simulink model "constant_rv_envTest"  (R2018b)
settings: Solver=FixedStepAuto  StartTime=0.0  StopTime=120  RelTol=1e-3  EnableMultiTasking=on
undefined symbols (not defined in the file or in its folder): attitude_estimation_lib, fswParams, simParams, t0, triad_coarse_estimator, TRIAD_coarse_estimator
libraries: vrlib x8, dspmathops x6, aerolibutil x5, magField_lib x2, time_Lib x2, solarPressure_lib x1, clock_lib x1, eclipseCheck x1, sunVector_lib x1, extended_kalman_filter_lib x1
settings Model: Creator=devantormey  LastModifiedBy=devantormey
settings OptimizationCC: LifeSpan=inf
settings DebuggingCC: SFUnexpectedBacktrackingDiag=warning  SFNoUnconditionalDefaultTransitionDiag=warning
settings SFSimCC: SimUseLocalCustomCode=off
settings RTWCC: RTWUseLocalCustomCode=off
settings CodeAppCC: StateflowObjectComments=on
settings GRTTargetCC: TargetLangStandard=C89/C90 (ANSI)  GeneratePreprocessorConditionals=Disable all
settings ConfigComp: CovMetricSettings=dw  CovHtmlReporting=on  CovSaveCumulativeToWorkspaceVar=on  CovSaveSingleToWorkspaceVar=on  CovExternalEMLEnable=off

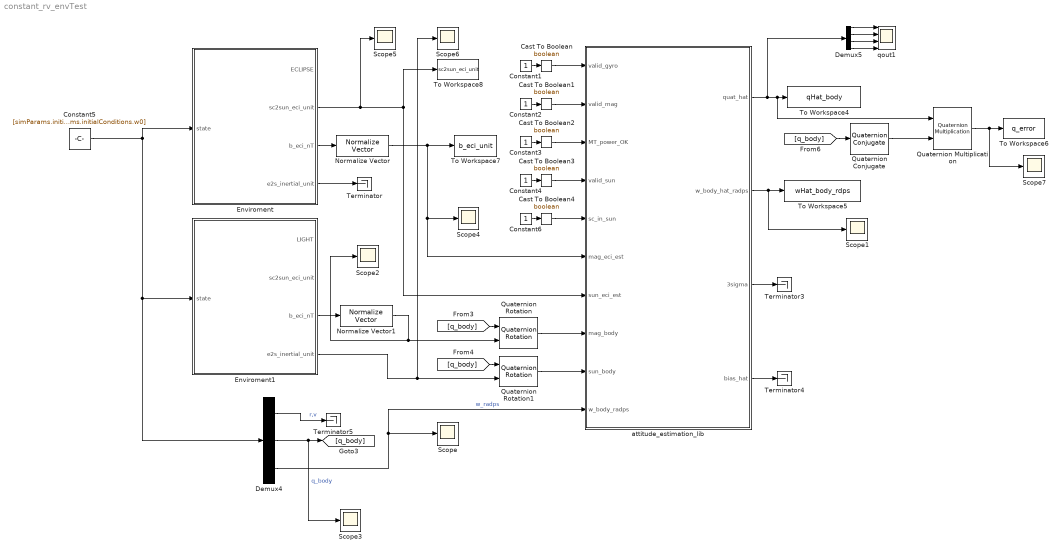
== system constant_rv_envTest ==
  Cast To Boolean{,1..4} (5 alike) : DataTypeConversion  OutDataTypeStr=boolean
  Constant{1..4,6} (5 alike) : Constant
  Constant5 : Constant  Value=[simParams.initialConditions.r0;simParams.initialConditions.v0;simParams.initialConditions.q0;simParams.initialConditions.w0]
  Demux4 : Demux  Outputs=[6 4 3]
  Demux5 : Demux
  Enviroment : Subsystem
  Enviroment1 : Subsystem
  Normalize Vector : vrlib/Utilities/Normalize Vector  maxzero=0
      settings: SourceProductName=Simulink 3D Animation  SourceProductBaseCode=VR
  Normalize Vector1 : vrlib/Utilities/Normalize Vector  maxzero=0
      settings: SourceProductName=Simulink 3D Animation  SourceProductBaseCode=VR
  Quaternion Conjugate : aerolibutil/Quaternion Conjugate
      settings: SourceProductName=Aerospace Blockset  SourceProductBaseCode=AE
  Quaternion Multiplication : aerolibutil/Quaternion Multiplication
  Quaternion Rotation : aerolibutil/Quaternion Rotation
  Quaternion Rotation1 : aerolibutil/Quaternion Rotation
  Scope{,1..7} (8 alike) : Scope
  Terminator{,3..5} (4 alike) : Terminator
  To Workspace4 : ToWorkspace  VariableName=qHat_body  SaveFormat=Timeseries  SampleTime=-1
  To Workspace5 : ToWorkspace  VariableName=wHat_body_rdps  SaveFormat=Timeseries  SampleTime=-1
  To Workspace6 : ToWorkspace  VariableName=q_error  SaveFormat=Timeseries  SampleTime=-1
  To Workspace7 : ToWorkspace  VariableName=b_eci_unit  SaveFormat=Timeseries  SampleTime=-1
  To Workspace8 : ToWorkspace  VariableName=sc2sun_eci_unit  SaveFormat=Timeseries  SampleTime=-1
  attitude_estimation_lib : Subsystem  AncestorBlock=attitude_estimation_lib/attitude_estimation_lib
  qout1 : Scope  NumInputPorts=4
  wires:
  attitude_estimation_lib/2(w_body_hat_radps) -> Scope1/1, To Workspace5/1
  attitude_estimation_lib/3(3sigma) -> Terminator3/1
  Constant1/1 -> Cast To Boolean/1
  Constant2/1 -> Cast To Boolean1/1
  Constant3/1 -> Cast To Boolean2/1
  Constant4/1 -> Cast To Boolean3/1
  Demux4/1 -> Terminator5/1  "r,v"
  Demux4/2 -> Scope3/1, [q_body]  "q_body"
  Normalize Vector1/1 -> Quaternion Rotation/2, Scope2/1
  [q_body] -> Quaternion Rotation/1
  [q_body] -> Quaternion Rotation1/1
  Enviroment1/4(e2s_inertial_unit) -> Quaternion Rotation1/2, Scope6/1
  Demux5/1 -> qout1/1
  Demux5/3 -> qout1/3
  Demux5/2 -> qout1/2
  Demux5/4 -> qout1/4
  Cast To Boolean/1 -> attitude_estimation_lib/1(valid_gyro)
  Cast To Boolean1/1 -> attitude_estimation_lib/2(valid_mag)
  Cast To Boolean2/1 -> attitude_estimation_lib/3(MT_power_OK)
  Cast To Boolean3/1 -> attitude_estimation_lib/4("valid_sun ")
  Cast To Boolean4/1 -> attitude_estimation_lib/5(sc_in_sun)
  Normalize Vector/1 -> Scope4/1, attitude_estimation_lib/6(mag_eci_est), To Workspace7/1
  Enviroment/2(sc2sun_eci_unit) -> Scope5/1, attitude_estimation_lib/7(sun_eci_est), To Workspace8/1
  Quaternion Rotation/1 -> attitude_estimation_lib/8(mag_body)
  Quaternion Rotation1/1 -> attitude_estimation_lib/9(sun_body)
  Demux4/3 -> attitude_estimation_lib/10(w_body_radps), Scope/1  "w_radps"
  attitude_estimation_lib/4(bias_hat) -> Terminator4/1
  attitude_estimation_lib/1(quat_hat) -> Demux5/1, Quaternion Multiplication/1, To Workspace4/1
  Enviroment/3(b_eci_nT) -> Normalize Vector/1
  Enviroment/4(e2s_inertial_unit) -> Terminator/1
  Quaternion Conjugate/1 -> Quaternion Multiplication/2
  [q_body] -> Quaternion Conjugate/1
  Quaternion Multiplication/1 -> Scope7/1, To Workspace6/1
  Enviroment1/3(b_eci_nT) -> Normalize Vector1/1
  Constant6/1 -> Cast To Boolean4/1
  Constant5/1 -> Demux4/1, Enviroment1/1(state), Enviroment/1(state)

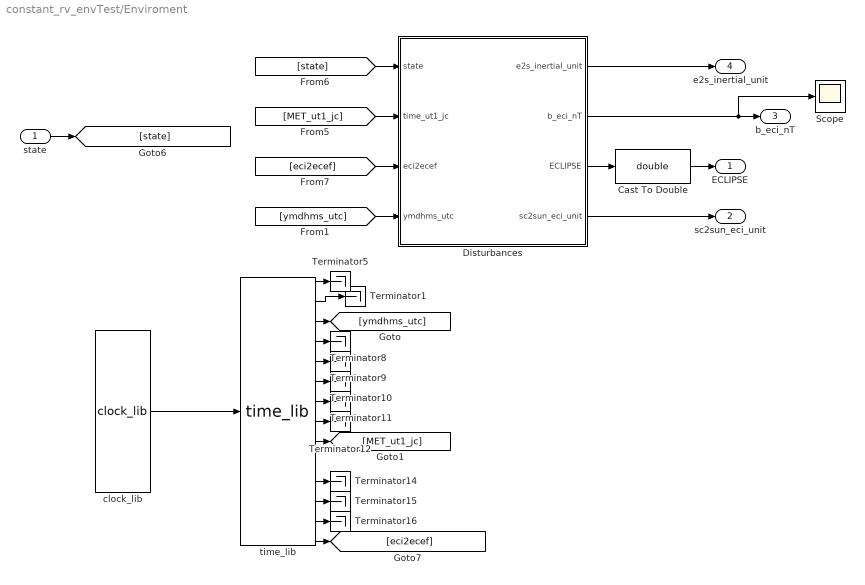
== system constant_rv_envTest/Enviroment ==
  state : Inport
  Cast To Double : DataTypeConversion  OutDataTypeStr=double
  Disturbances : Subsystem
  Scope : Scope
  Terminator{1,5,8..12,14..16} (10 alike) : Terminator
  clock_lib : clock_lib/clock_lib  SystemSampleTime=-1
  "time_lib " : time_Lib/time_lib    SystemSampleTime=-1
  ECLIPSE : Outport
  sc2sun_eci_unit : Outport  Port=2
  b_eci_nT : Outport  Port=3
  e2s_inertial_unit : Outport  Port=4
  wires:
  state/1 -> [state]
  clock_lib/1 -> "time_lib "/1
  "time_lib "/14 -> [eci2ecef]
  [eci2ecef] -> Disturbances/3(eci2ecef)
  [MET_ut1_jc] -> Disturbances/2(time_ut1_jc)
  [state] -> Disturbances/1(state)
  Cast To Double/1 -> ECLIPSE/1
  Disturbances/3(ECLIPSE) -> Cast To Double/1
  "time_lib "/1 -> Terminator5/1
  "time_lib "/2 -> Terminator1/1
  "time_lib "/3 -> [ymdhms_utc]
  "time_lib "/4 -> Terminator8/1
  "time_lib "/5 -> Terminator9/1
  "time_lib "/6 -> Terminator10/1
  "time_lib "/7 -> Terminator11/1
  "time_lib "/8 -> Terminator12/1
  "time_lib "/9 -> [MET_ut1_jc]
  "time_lib "/11 -> Terminator14/1
  "time_lib "/12 -> Terminator15/1
  "time_lib "/13 -> Terminator16/1
  [ymdhms_utc] -> Disturbances/4(ymdhms_utc)
  Disturbances/4(sc2sun_eci_unit) -> sc2sun_eci_unit/1
  Disturbances/2(b_eci_nT) -> Scope/1, b_eci_nT/1
  Disturbances/1(e2s_inertial_unit) -> e2s_inertial_unit/1

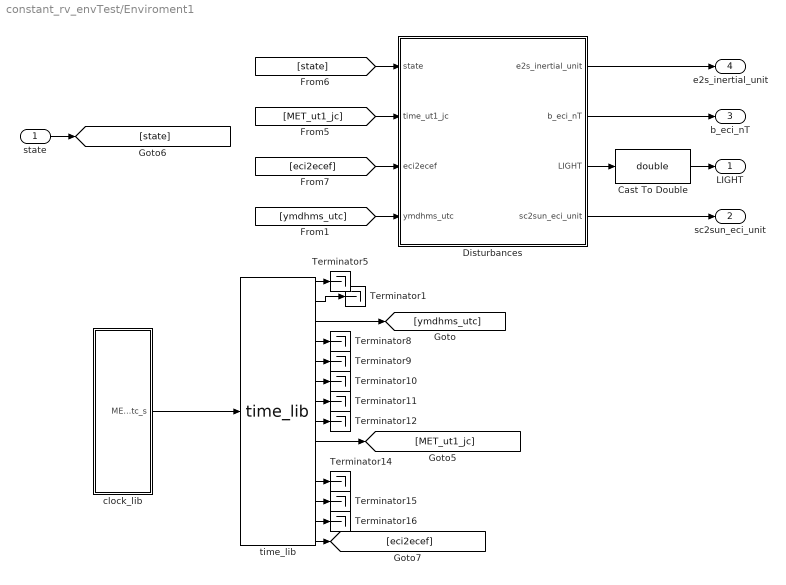
== system constant_rv_envTest/Enviroment1 ==
  state : Inport
  Cast To Double : DataTypeConversion  OutDataTypeStr=double
  Disturbances : Subsystem
  Terminator{1,5,8..12,14..16} (10 alike) : Terminator
  clock_lib : Subsystem  AncestorBlock=clock_lib/clock_lib
  "time_lib " : time_Lib/time_lib    SystemSampleTime=-1
  LIGHT : Outport
  sc2sun_eci_unit : Outport  Port=2
  b_eci_nT : Outport  Port=3
  e2s_inertial_unit : Outport  Port=4
  wires:
  state/1 -> [state]
  clock_lib/1(MET_utc_s) -> "time_lib "/1
  "time_lib "/14 -> [eci2ecef]
  [eci2ecef] -> Disturbances/3(eci2ecef)
  [MET_ut1_jc] -> Disturbances/2(time_ut1_jc)
  [state] -> Disturbances/1(state)
  Cast To Double/1 -> LIGHT/1
  Disturbances/3(LIGHT) -> Cast To Double/1
  "time_lib "/1 -> Terminator5/1
  "time_lib "/2 -> Terminator1/1
  "time_lib "/3 -> [ymdhms_utc]
  "time_lib "/4 -> Terminator8/1
  "time_lib "/5 -> Terminator9/1
  "time_lib "/6 -> Terminator10/1
  "time_lib "/7 -> Terminator11/1
  "time_lib "/8 -> Terminator12/1
  "time_lib "/9 -> [MET_ut1_jc]
  "time_lib "/11 -> Terminator14/1
  "time_lib "/12 -> Terminator15/1
  "time_lib "/13 -> Terminator16/1
  [ymdhms_utc] -> Disturbances/4(ymdhms_utc)
  Disturbances/4(sc2sun_eci_unit) -> sc2sun_eci_unit/1
  Disturbances/2(b_eci_nT) -> b_eci_nT/1
  Disturbances/1(e2s_inertial_unit) -> e2s_inertial_unit/1

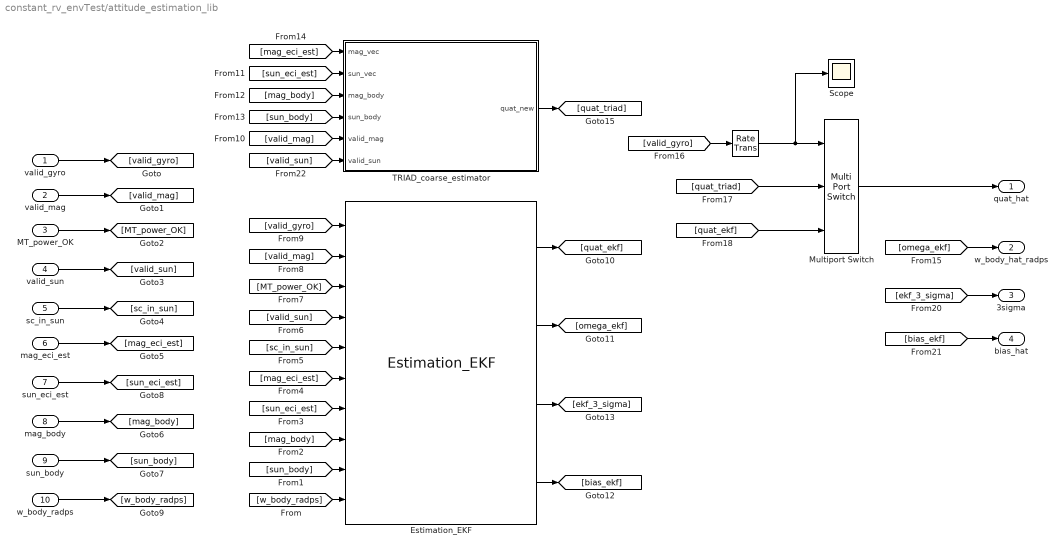
== system constant_rv_envTest/attitude_estimation_lib ==
  valid_gyro : Inport
  valid_mag : Inport  Port=2
  MT_power_OK : Inport  Port=3
  "valid_sun " : Inport  Port=4
  sc_in_sun : Inport  Port=5
  mag_eci_est : Inport  Port=6
  sun_eci_est : Inport  Port=7
  mag_body : Inport  Port=8
  sun_body : Inport  Port=9
  w_body_radps : Inport  Port=10
  " " : RateTransition  InitialCondition=fswParams.estimation.ic.rt_valid_gyro  OutPortSampleTime=fswParams.estimation.sample_time_s
  "Estimation_EKF " : extended_kalman_filter_lib/Estimation_EKF   SystemSampleTime=-1
      link override " ": InitialCondition=fswParams.estimation.ic.rt_valid_gyro
  Multiport Switch : MultiPortSwitch  DataPortOrder=Zero-based contiguous  Inputs=2  zeroidx=on
  Scope : Scope
  TRIAD_coarse_estimator : Subsystem  AncestorBlock=triad_coarse_estimator/TRIAD_coarse_estimator
  quat_hat : Outport
  w_body_hat_radps : Outport  Port=2
  3sigma : Outport  Port=3
  bias_hat : Outport  Port=4
  wires:
  Multiport Switch/1 -> quat_hat/1
  [quat_ekf] -> Multiport Switch/3
  [quat_triad] -> Multiport Switch/2
  " "/1 -> Scope/1, Multiport Switch/1
  "Estimation_EKF "/2 -> [omega_ekf]
  "Estimation_EKF "/3 -> [ekf_3_sigma]
  "Estimation_EKF "/4 -> [bias_ekf]
  [valid_gyro] -> " "/1
  "Estimation_EKF "/1 -> [quat_ekf]
  TRIAD_coarse_estimator/1(quat_new) -> [quat_triad]
  [valid_sun] -> TRIAD_coarse_estimator/6(valid_sun)
  [valid_mag] -> TRIAD_coarse_estimator/5(valid_mag)
  [sun_body] -> TRIAD_coarse_estimator/4(sun_body)
  [mag_body] -> TRIAD_coarse_estimator/3(mag_body)
  [sun_eci_est] -> TRIAD_coarse_estimator/2("sun_vec ")
  [mag_eci_est] -> TRIAD_coarse_estimator/1("mag_vec ")
  [w_body_radps] -> "Estimation_EKF "/10
  w_body_radps/1 -> [w_body_radps]
  [sun_body] -> "Estimation_EKF "/9
  [mag_body] -> "Estimation_EKF "/8
  [sun_eci_est] -> "Estimation_EKF "/7
  [mag_eci_est] -> "Estimation_EKF "/6
  [sc_in_sun] -> "Estimation_EKF "/5
  [valid_sun] -> "Estimation_EKF "/4
  [MT_power_OK] -> "Estimation_EKF "/3
  [valid_mag] -> "Estimation_EKF "/2
  [valid_gyro] -> "Estimation_EKF "/1
  sun_eci_est/1 -> [sun_eci_est]
  mag_eci_est/1 -> [mag_eci_est]
  sc_in_sun/1 -> [sc_in_sun]
  [omega_ekf] -> w_body_hat_radps/1
  [ekf_3_sigma] -> 3sigma/1
  [bias_ekf] -> bias_hat/1
  MT_power_OK/1 -> [MT_power_OK]
  sun_body/1 -> [sun_body]
  mag_body/1 -> [mag_body]
  "valid_sun "/1 -> [valid_sun]
  valid_mag/1 -> [valid_mag]
  valid_gyro/1 -> [valid_gyro]

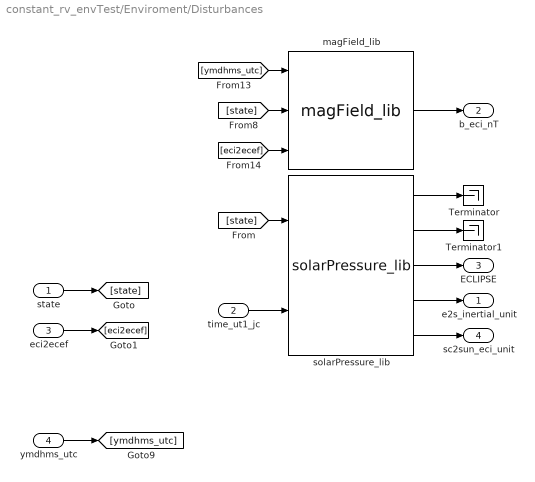
== system constant_rv_envTest/Enviroment/Disturbances ==
  state : Inport
  time_ut1_jc : Inport  Port=2
  eci2ecef : Inport  Port=3
  ymdhms_utc : Inport  Port=4
  Terminator : Terminator
  Terminator1 : Terminator
  magField_lib : magField_lib/magField_lib  SystemSampleTime=-1
  solarPressure_lib : solarPressure_lib/solarPressure_lib  SystemSampleTime=-1
  e2s_inertial_unit : Outport
  b_eci_nT : Outport  Port=2
  ECLIPSE : Outport  Port=3
  sc2sun_eci_unit : Outport  Port=4
  wires:
  solarPressure_lib/3 -> ECLIPSE/1
  solarPressure_lib/1 -> Terminator/1
  solarPressure_lib/4 -> e2s_inertial_unit/1
  solarPressure_lib/2 -> Terminator1/1
  time_ut1_jc/1 -> solarPressure_lib/2
  state/1 -> [state]
  [state] -> solarPressure_lib/1
  eci2ecef/1 -> [eci2ecef]
  [state] -> magField_lib/2
  ymdhms_utc/1 -> [ymdhms_utc]
  [ymdhms_utc] -> magField_lib/1
  [eci2ecef] -> magField_lib/3
  solarPressure_lib/5 -> sc2sun_eci_unit/1
  magField_lib/1 -> b_eci_nT/1

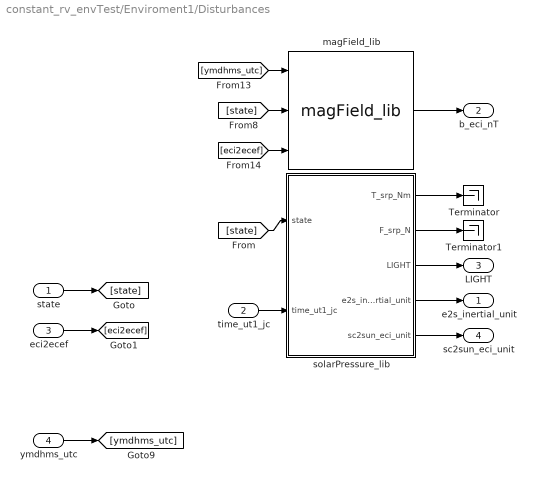
== system constant_rv_envTest/Enviroment1/Disturbances ==
  state : Inport
  time_ut1_jc : Inport  Port=2
  eci2ecef : Inport  Port=3
  ymdhms_utc : Inport  Port=4
  Terminator : Terminator
  Terminator1 : Terminator
  magField_lib : magField_lib/magField_lib  SystemSampleTime=-1
      link override Rate Transition2: InitialCondition=0
  solarPressure_lib : Subsystem  AncestorBlock=solarPressure_lib/solarPressure_lib
  e2s_inertial_unit : Outport
  b_eci_nT : Outport  Port=2
  LIGHT : Outport  Port=3
  sc2sun_eci_unit : Outport  Port=4
  wires:
  solarPressure_lib/3(LIGHT) -> LIGHT/1
  solarPressure_lib/1(T_srp_Nm) -> Terminator/1
  solarPressure_lib/4(e2s_inertial_unit) -> e2s_inertial_unit/1
  solarPressure_lib/2(F_srp_N) -> Terminator1/1
  time_ut1_jc/1 -> solarPressure_lib/2(time_ut1_jc)
  state/1 -> [state]
  [state] -> solarPressure_lib/1(state)
  eci2ecef/1 -> [eci2ecef]
  [state] -> magField_lib/2
  ymdhms_utc/1 -> [ymdhms_utc]
  [ymdhms_utc] -> magField_lib/1
  [eci2ecef] -> magField_lib/3
  magField_lib/1 -> b_eci_nT/1
  solarPressure_lib/5(sc2sun_eci_unit) -> sc2sun_eci_unit/1

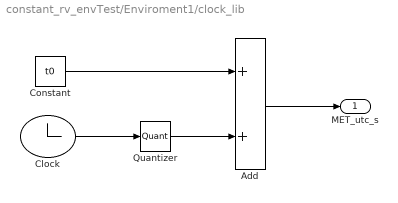
== system constant_rv_envTest/Enviroment1/clock_lib ==
  Add : Sum
  Clock : Clock
  Constant : Constant  Value=t0
  Quantizer : Quantizer  QuantizationInterval=simParams.time.res
  MET_utc_s : Outport
  wires:
  Add/1 -> MET_utc_s/1
  Quantizer/1 -> Add/2
  Constant/1 -> Add/1
  Clock/1 -> Quantizer/1

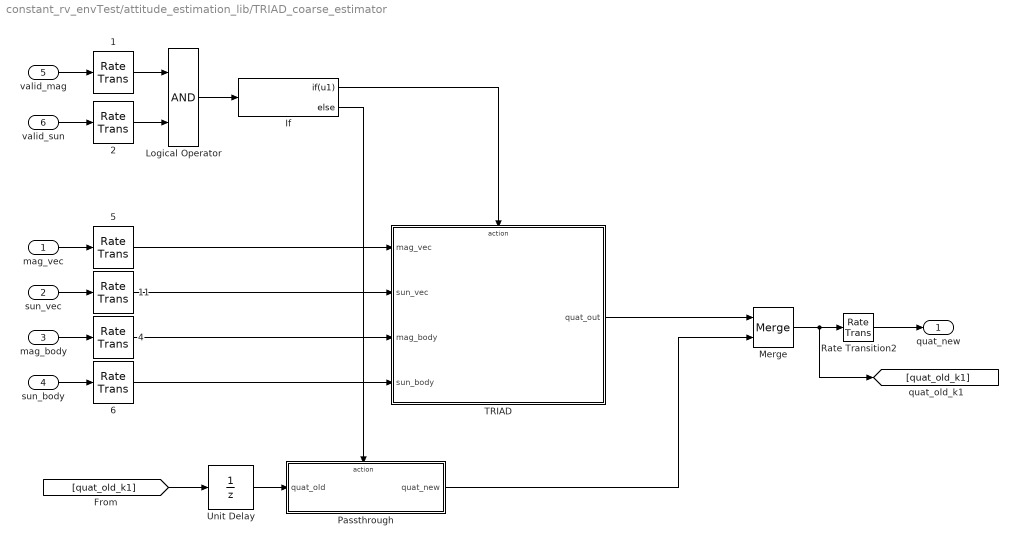
== system constant_rv_envTest/attitude_estimation_lib/TRIAD_coarse_estimator ==
  "mag_vec " : Inport
  "sun_vec " : Inport  Port=2
  mag_body : Inport  Port=3
  sun_body : Inport  Port=4
  valid_mag : Inport  Port=5
  valid_sun : Inport  Port=6
  " 1" : RateTransition  InitialCondition=fswParams.estimation.ic.rt_valid_mag  OutPortSampleTime=fswParams.estimation.sample_time_s
  " 11" : RateTransition  InitialCondition=fswParams.estimation.ic.rt_sun_eci_est  OutPortSampleTime=fswParams.estimation.sample_time_s
  " 2" : RateTransition  InitialCondition=fswParams.estimation.ic.rt_valid_sun  OutPortSampleTime=fswParams.estimation.sample_time_s
  " 4" : RateTransition  InitialCondition=fswParams.estimation.ic.rt_mag_body  OutPortSampleTime=fswParams.estimation.sample_time_s
  " 5" : RateTransition  InitialCondition=fswParams.estimation.ic.rt_mag_eci_est  OutPortSampleTime=fswParams.estimation.sample_time_s
  " 6" : RateTransition  InitialCondition=fswParams.estimation.ic.rt_sun_body  OutPortSampleTime=fswParams.estimation.sample_time_s
  If : If  IfExpression=u1
  Logical Operator : Logic  AllPortsSameDT=off  OutDataTypeStr=boolean
  Merge : Merge
  Passthrough : Subsystem  TreatAsAtomicUnit=on
  Rate Transition2 : RateTransition  InitialCondition=fswParams.estimation.ic.quat_est_init
  "TRIAD " : Subsystem  TreatAsAtomicUnit=on
  Unit Delay : UnitDelay  InitialCondition=fswParams.estimation.ic.quat_est_init  SampleTime=fswParams.estimation.sample_time_s
  quat_new : Outport
  wires:
  Unit Delay/1 -> Passthrough/1(quat_old)
  [quat_old_k1] -> Unit Delay/1
  " 5"/1 -> "TRIAD "/1("mag_vec ")
  " 11"/1 -> "TRIAD "/2("sun_vec ")
  " 6"/1 -> "TRIAD "/4(sun_body)
  " 4"/1 -> "TRIAD "/3(mag_body)
  " 2"/1 -> Logical Operator/2
  " 1"/1 -> Logical Operator/1
  Rate Transition2/1 -> quat_new/1
  Logical Operator/1 -> If/1
  valid_sun/1 -> " 2"/1
  valid_mag/1 -> " 1"/1
  Merge/1 -> Rate Transition2/1, [quat_old_k1]
  Passthrough/1(quat_new) -> Merge/2
  "TRIAD "/1("quat_out ") -> Merge/1
  If/2 -> Passthrough/Action
  If/1 -> "TRIAD "/Action
  sun_body/1 -> " 6"/1
  mag_body/1 -> " 4"/1
  "sun_vec "/1 -> " 11"/1
  "mag_vec "/1 -> " 5"/1

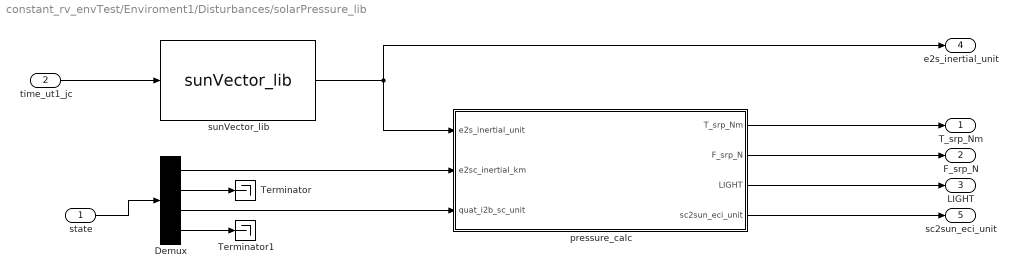
== system constant_rv_envTest/Enviroment1/Disturbances/solarPressure_lib ==
  state : Inport
  time_ut1_jc : Inport  Port=2
  Demux : Demux  Outputs=[3 3 4 3]
  Terminator : Terminator
  Terminator1 : Terminator
  pressure_calc : Subsystem
  sunVector_lib : sunVector_lib/sunVector_lib  SystemSampleTime=-1
  T_srp_Nm : Outport
  F_srp_N : Outport  Port=2
  LIGHT : Outport  Port=3
  e2s_inertial_unit : Outport  Port=4
  sc2sun_eci_unit : Outport  Port=5
  wires:
  pressure_calc/3(LIGHT) -> LIGHT/1
  state/1 -> Demux/1
  Demux/4 -> Terminator1/1
  time_ut1_jc/1 -> sunVector_lib/1
  Demux/1 -> pressure_calc/2(e2sc_inertial_km)
  Demux/2 -> Terminator/1
  Demux/3 -> pressure_calc/3(quat_i2b_sc_unit)
  pressure_calc/1(T_srp_Nm) -> T_srp_Nm/1
  sunVector_lib/1 -> e2s_inertial_unit/1, pressure_calc/1(e2s_inertial_unit)
  pressure_calc/2(F_srp_N) -> F_srp_N/1
  pressure_calc/4(sc2sun_eci_unit) -> sc2sun_eci_unit/1

== system constant_rv_envTest/attitude_estimation_lib/TRIAD_coarse_estimator/Passthrough ==
  quat_old : Inport
  Action Port : ActionPort  ActionType=else
  quat_new : Outport
  wires:
  quat_old/1 -> quat_new/1

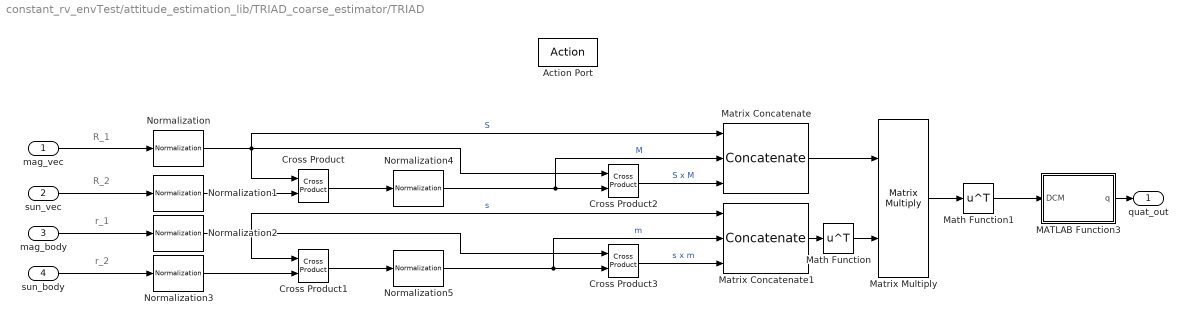
== system constant_rv_envTest/attitude_estimation_lib/TRIAD_coarse_estimator/TRIAD  ==
  note: r_1
  note: r_2
  note: R_1
  note: R_2
  "mag_vec " : Inport
  "sun_vec " : Inport  Port=2
  mag_body : Inport  Port=3
  sun_body : Inport  Port=4
  Action Port : ActionPort  ActionType=then
  Cross Product{,1..3} (4 alike) : vrlib/Utilities/Cross Product
      settings: SourceProductBaseCode=VR
  MATLAB Function3 : MATLAB Function  TreatAsAtomicUnit=on
  Math Function : Math  Operator=transpose  SaturateOnIntegerOverflow=on
  Math Function1 : Math  Operator=transpose  SaturateOnIntegerOverflow=on
  Matrix Concatenate : Concatenate  NumInputs=3  Mode=Multidimensional array  ConcatenateDimension=2
  Matrix Concatenate1 : Concatenate  NumInputs=3  Mode=Multidimensional array  ConcatenateDimension=2
  Matrix Multiply : Product  Multiplication=Matrix(*)
  Normalization{,1..5} (6 alike) : dspmathops/Normalization  NormType=2-norm  Bias=1e-10  NormOver=Each column  Dimension=1  roundingMode=Floor  overflowMode=off  accumDataTypeStr=Inherit: Same as product output  accumLastDataTypeStr=Inherit: Same as product output  outputDataTypeStr=Inherit: Same as product output  outputMin=[]  outputMax=[]  outputLastDataTypeStr=Inherit: Same as product output
      settings: SourceProductName=DSP System Toolbox
  "quat_out " : Outport
  wires:
  Normalization/1 -> Cross Product2/1, Cross Product/1, Matrix Concatenate/1  "S"
  Matrix Multiply/1 -> Math Function1/1
  MATLAB Function3/1(q) -> "quat_out "/1
  Math Function/1 -> Matrix Multiply/2
  Matrix Concatenate/1 -> Matrix Multiply/1
  Matrix Concatenate1/1 -> Math Function/1
  Cross Product3/1 -> Matrix Concatenate1/3  "s x m"
  Cross Product2/1 -> Matrix Concatenate/3  "S x M"
  Normalization5/1 -> Cross Product3/2, Matrix Concatenate1/2  "m"
  Normalization4/1 -> Cross Product2/2, Matrix Concatenate/2  "M"
  Cross Product1/1 -> Normalization5/1
  Cross Product/1 -> Normalization4/1
  Normalization3/1 -> Cross Product1/2
  Normalization2/1 -> Cross Product1/1, Cross Product3/1, Matrix Concatenate1/1  "s"
  Normalization1/1 -> Cross Product/2
  sun_body/1 -> Normalization3/1
  mag_body/1 -> Normalization2/1
  "sun_vec "/1 -> Normalization1/1
  "mag_vec "/1 -> Normalization/1
  Math Function1/1 -> MATLAB Function3/1(DCM)

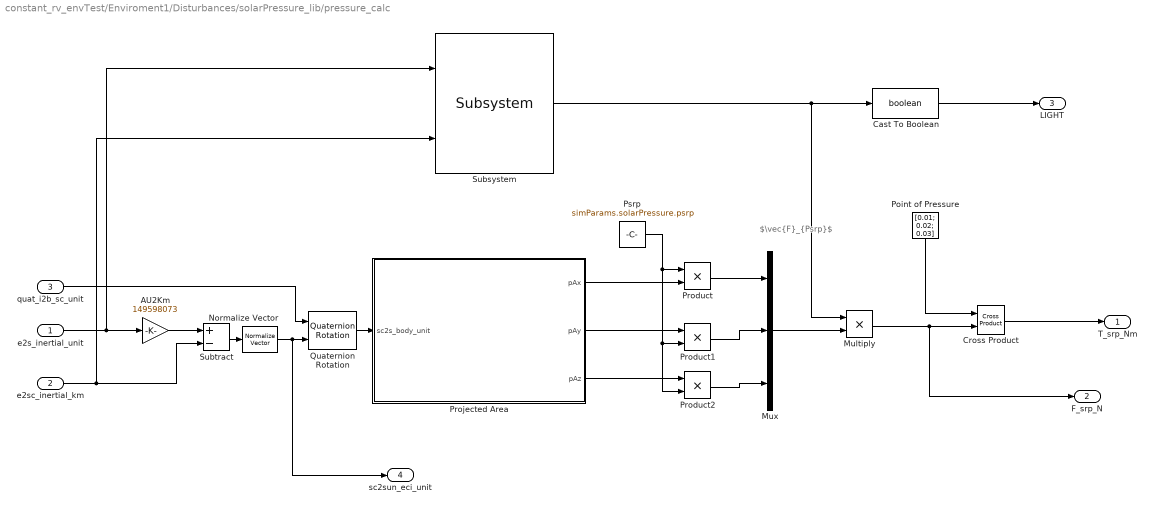
== system constant_rv_envTest/Enviroment1/Disturbances/solarPressure_lib/pressure_calc ==
  note: $\vec{F}_{Psrp}$
  e2s_inertial_unit : Inport
  e2sc_inertial_km : Inport  Port=2
  quat_i2b_sc_unit : Inport  Port=3
  AU2Km : Gain  Gain=149598073
  Cast To Boolean : DataTypeConversion  OutDataTypeStr=boolean
  Cross Product : vrlib/Utilities/Cross Product
      settings: SourceProductBaseCode=VR
  Multiply : Product
  Mux : Mux  Inputs=3
  Normalize Vector : vrlib/Utilities/Normalize Vector  maxzero=0
      settings: SourceProductName=Simulink 3D Animation  SourceProductBaseCode=VR
  Point of Pressure : Constant  Value=[0.01; 0.02; 0.03]
  Product : Product
  Product1 : Product
  Product2 : Product
  Projected Area : Subsystem
  Psrp : Constant  Value=simParams.solarPressure.psrp
  Quaternion Rotation : aerolibutil/Quaternion Rotation
  Subsystem : eclipseCheck/Subsystem  SystemSampleTime=-1
  Subtract : Sum  Inputs=+-
  T_srp_Nm : Outport
  F_srp_N : Outport  Port=2
  LIGHT : Outport  Port=3
  sc2sun_eci_unit : Outport  Port=4
  wires:
  Normalize Vector/1 -> sc2sun_eci_unit/1, Quaternion Rotation/2
  Subtract/1 -> Normalize Vector/1
  AU2Km/1 -> Subtract/1
  Cast To Boolean/1 -> LIGHT/1
  Subsystem/1 -> Multiply/1, Cast To Boolean/1
  Multiply/1 -> Cross Product/2, F_srp_N/1
  Mux/1 -> Multiply/2
  Quaternion Rotation/1 -> Projected Area/1(sc2s_body_unit)
  quat_i2b_sc_unit/1 -> Quaternion Rotation/1
  e2sc_inertial_km/1 -> Subsystem/2, Subtract/2
  e2s_inertial_unit/1 -> Subsystem/1, AU2Km/1
  Cross Product/1 -> T_srp_Nm/1
  Point of Pressure/1 -> Cross Product/1
  Product2/1 -> Mux/3
  Product1/1 -> Mux/2
  Product/1 -> Mux/1
  Projected Area/3(pAz) -> Product2/1
  Projected Area/2(pAy) -> Product1/1
  Psrp/1 -> Product/1, Product1/2, Product2/2
  Projected Area/1(pAx) -> Product/2

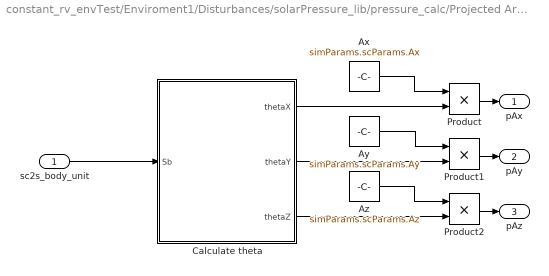
== system constant_rv_envTest/Enviroment1/Disturbances/solarPressure_lib/pressure_calc/Projected Area ==
  sc2s_body_unit : Inport
  Ax : Constant  Value=simParams.scParams.Ax
  Ay : Constant  Value=simParams.scParams.Ay
  Az : Constant  Value=simParams.scParams.Az
  Calculate theta : MATLAB Function  TreatAsAtomicUnit=on
  Product : Product
  Product1 : Product
  Product2 : Product
  pAx : Outport
  pAy : Outport  Port=2
  pAz : Outport  Port=3
  wires:
  Ax/1 -> Product/1
  sc2s_body_unit/1 -> Calculate theta/1(Sb)
  Product/1 -> pAx/1
  Calculate theta/2(thetaY) -> Product1/2
  Calculate theta/1(thetaX) -> Product/2
  Ay/1 -> Product1/1
  Calculate theta/3(thetaZ) -> Product2/2
  Az/1 -> Product2/1
  Product2/1 -> pAz/1
  Product1/1 -> pAy/1

== matlab function constant_rv_envTest/Enviroment1/Disturbances/solarPressure_lib/pressure_calc/Projected Area/Calculate theta ==
  data: Sb input; thetaX output; thetaY output; thetaZ output
% Author: Devan Tormey
% Date: 2/21/2019
function [thetaX,thetaY,thetaZ] = fcn(Sb)
% Description: This function computes the dot product of the sun vector
% with the appropriate body coordinate vector.
%~~~~~~~~~~~~~ 
%  Variables 
%~~~~~~~~~~~~~~
% Sb - this is the sun vector (calculated elsewhere)
% ThetaXYZ - as these are all unit vectors the dot product produces the
% cosine of the angle in between

    if Sb(1) >= 0 
        thetaX = dot(Sb,[1;0;0]);
    else 
        thetaX = dot(Sb,[-1;0;0]);
    end

    if Sb(2) >= 0 
        thetaY = dot(Sb,[0;1;0]);
    else 
        thetaY = dot(Sb,[0;-1;0]);
    end

    if Sb(3) >= 0 
        thetaZ = dot(Sb,[0;0;1]);
    else 
        thetaZ = dot(Sb,[0;0;-1]);
    end

end

== matlab function constant_rv_envTest/attitude_estimation_lib/TRIAD_coarse_estimator/TRIAD /MATLAB Function3 ==
  data: DCM input; q output
function q = myDCM2quat( DCM )
% ----------------------------------------------------------------------- %
% UW HuskySat-1, ADCS Team
%
% DCM to Quaternion conversion assuming positive scalar part
%
% T. Reynolds 1.15.18
% #codegen
% ----------------------------------------------------------------------- %
q   = zeros(4,1);

tr  = trace(DCM);

q(1)    = 0.5*sqrt(tr + 1);

if( q(1) ~= 0 )
    eta     = 1/(4*q(1));
    q(2)    = eta*(DCM(2,3) - DCM(3,2));
    q(3)    = eta*(DCM(3,1) - DCM(1,3));
    q(4)    = eta*(DCM(1,2) - DCM(2,1));
else
    q(2)  = sqrt(0.5*(DCM(1,1) + 1));
    q(3)  = sign(DCM(1,2))*sqrt(0.5*(DCM(2,2) + 1));
    q(4)  = sign(DCM(1,3))*sqrt(0.5*(DCM(3,3) + 1));
end


end
